simulink model "course_loop"  (R2020a)
settings: Solver=VariableStepAuto  StartTime=0.0  StopTime=300  RelTol=1e-3
undefined symbols (not defined in the file or in its folder): AP, trans_func
libraries: slctrlblks x2
settings Model: Creator=nikhil  LastModifiedBy=VTOL_HYD
settings SFSimCC: CustomCodeUndefinedFunction=UseInterfaceOnly

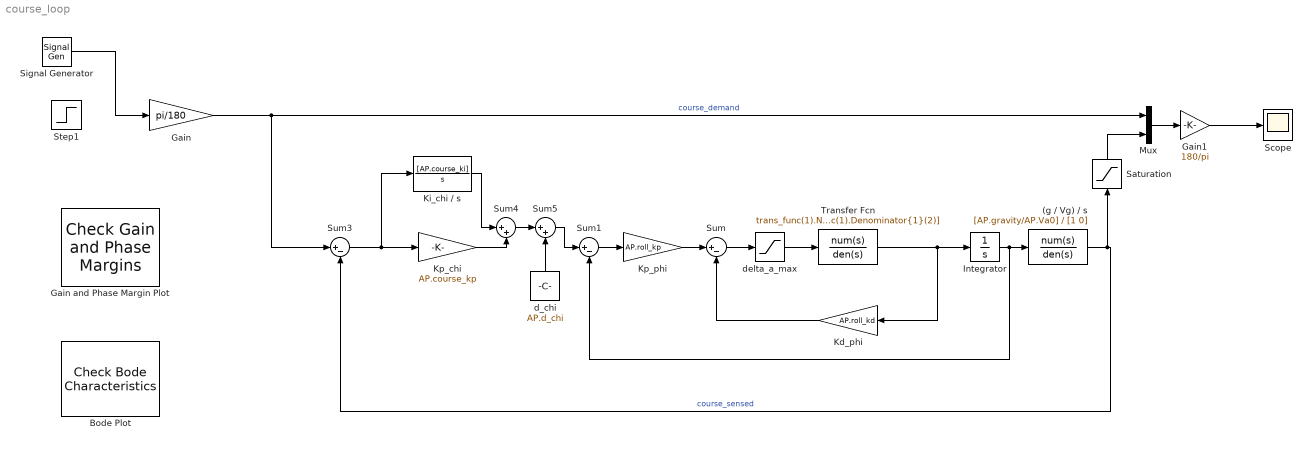
== system course_loop ==
  (g / Vg) / s : TransferFcn  Numerator=[AP.gravity/AP.Va0]  Denominator=[1 0]
  Bode Plot : slctrlblks/Model Verification/Check Bode  Characteristics  InstantiateOnLoad=on  SaveOperatingPoints=off  LinearizationIOs={'/Gain', 1, 'in', 'off', '';'/Saturation', 1, 'out', 'on', ''}  LinearizeAt=SnapshotTimes  SnapshotTimes=[0]  TriggerType=rising  SampleTime=auto  RateConversionMethod=zoh  PreWarpFreq=10  UseExactDelayModel=off  UseFullBlockNameLabels=off  UseBusSignalLabels=off  enabled=on  stopWhenAssertionFail=off  export=off  ViewDlgPos=[753 213 1065 602]  OpenViewOnLoad=off  LaunchViewOnOpen=off  FrequencyUnits=rad/s  MagnitudeUnits=dB  PhaseUnits=deg  TimeUnits=seconds  EnableUpperBound=off  UpperBoundFrequencies=[]  UpperBoundMagnitudes=[]  EnableLowerBound=off  LowerBoundFrequencies=[]  LowerBoundMagnitudes=[]
  Gain : Gain  Gain=pi/180
  Gain and Phase Margin Plot : slctrlblks/Model Verification/Check Gain and Phase Margins  InstantiateOnLoad=on  SaveOperatingPoints=off  LinearizationIOs={'/Gain', 1, 'in', 'off', '';'/Saturation', 1, 'out', 'on', ''}  LinearizeAt=SnapshotTimes  SnapshotTimes=[0]  TriggerType=rising  SampleTime=auto  RateConversionMethod=zoh  PreWarpFreq=10  UseExactDelayModel=off  UseFullBlockNameLabels=off  UseBusSignalLabels=off  enabled=on  stopWhenAssertionFail=off  export=off  ViewDlgPos=[1 41 1920 963]  LaunchViewOnOpen=off  OpenViewOnLoad=off  FrequencyUnits=rad/s  MagnitudeUnits=dB  PhaseUnits=deg  TimeUnits=seconds  EnableMargins=off  GainMargin=[]  PhaseMargin=[]  PlotType=nyquist  FeedbackSign=-1
      settings: SourceProductBaseCode=SD  SaveToWorkspace=off  SaveName=sys
  Gain1 : Gain  Gain=180/pi
  Integrator : Integrator
  Kd_phi : Gain  Gain=AP.roll_kd
  Ki_chi / s : TransferFcn  Numerator=[AP.course_ki]  Denominator=[1 0]
  Kp_chi : Gain  Gain=AP.course_kp
  Kp_phi : Gain  Gain=AP.roll_kp
  Mux : Mux  Inputs=2
  Saturation : Saturate  UpperLimit=7  LowerLimit=-7
  Scope : Scope
  Signal Generator : SignalGenerator  Amplitude=110  Frequency=.09  Units=rad/sec
  Step1 : Step  After=200  SampleTime=5
  Sum : Sum  Inputs=|+-
  Sum1 : Sum  Inputs=|+-
  Sum3 : Sum  Inputs=|+-
  Sum4 : Sum  Inputs=|++
  Sum5 : Sum  Inputs=|++
  Transfer Fcn : TransferFcn  Numerator=trans_func(1).Numerator{1}  Denominator=[trans_func(1).Denominator{1}(1), trans_func(1).Denominator{1}(2)]
  d_chi : Constant  Value=AP.d_chi
  delta_a_max : Saturate  UpperLimit=0.785  LowerLimit=-.785
  wires:
  Transfer Fcn/1 -> Kd_phi/1, Integrator/1
  Kd_phi/1 -> Sum/2
  Gain/1 -> Sum3/1, Mux/1  "course_demand"
  Sum1/1 -> Kp_phi/1
  Kp_phi/1 -> Sum/1
  (g / Vg) / s/1 -> Sum3/2, Saturation/1  "course_sensed"
  Sum3/1 -> Ki_chi / s/1, Kp_chi/1
  Ki_chi / s/1 -> Sum4/1
  Kp_chi/1 -> Sum4/2
  Saturation/1 -> Mux/2
  Mux/1 -> Gain1/1
  Gain1/1 -> Scope/1
  Sum/1 -> delta_a_max/1
  delta_a_max/1 -> Transfer Fcn/1
  Integrator/1 -> (g / Vg) / s/1, Sum1/2
  d_chi/1 -> Sum5/2
  Sum4/1 -> Sum5/1
  Sum5/1 -> Sum1/1
  Signal Generator/1 -> Gain/1
